simulink model "missile"  (R2018b)
settings: Solver=ode4  StartTime=0.0  StopTime=inf  FixedStep=0.03  RelTol=1e-3
values from neighbouring files (symbols this model uses):
  g = 9.8    [init.m]
  GP_switch = 1    [init.m]
  halfa_seeker_lock = 15    [init.m]
  init_m = [0 5000 0 180 0 deg2rad(0)]    [init.m]
  K = 3.5    [init.m]
  mass = [200 170 130]    [init.m]
  nn_lim = 40    [init.m]
  r_seeker_active = 20000    [init.m]
  S = 0.03    [init.m]
  TGO_max = 200    [init.m]
  thrust = [40000 20000 0]    [init.m]
  thrust_time_idx = [0 4 12]    [init.m]
undefined symbols (not defined in the file or in its folder): CD0, CDi, CL_idx, CLmax, ma_idx
libraries: aerolibasang x2, sharedutil x1, aerolibatmos2 x1, aerolibconvert2 x1
settings Model: Creator=niao4  LastModifiedBy=ysq
settings RTWCC: TargetLang=C++
settings GRTTargetCC: TargetLangStandard=C++03 (ISO)  MatFileLogging=off  MultiInstanceERTCode=on  CodeInterfacePackaging=C++ class

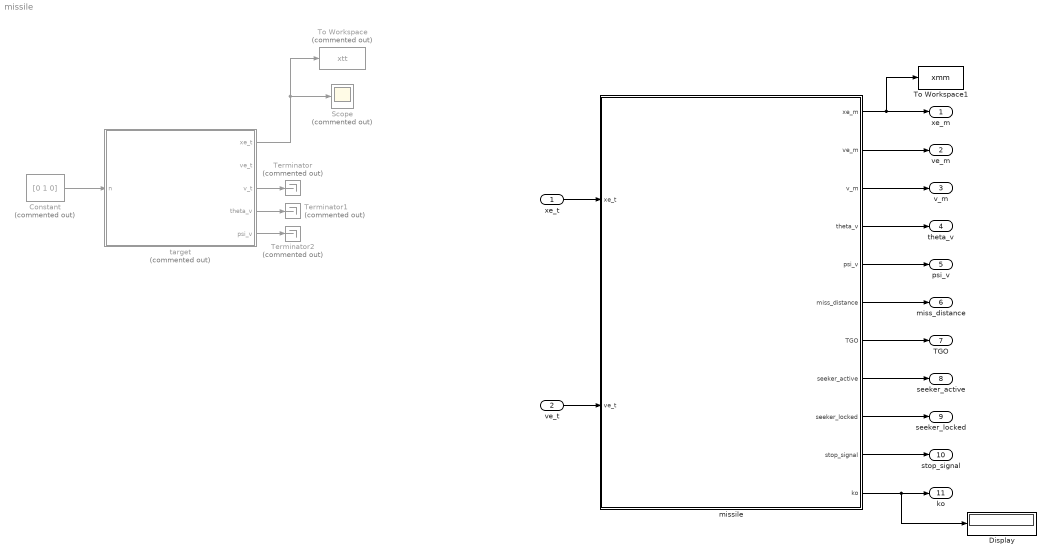
== system missile ==
  xe_t : Inport
  ve_t : Inport  Port=2
  Constant : Constant  Commented=on  Value=[0 1 0]
  Display : Display
  Scope : Scope  Commented=on
  Terminator : Terminator  Commented=on
  Terminator1 : Terminator  Commented=on
  Terminator2 : Terminator  Commented=on
  To Workspace : ToWorkspace  Commented=on  VariableName=xtt  SampleTime=-1
  To Workspace1 : ToWorkspace  VariableName=xmm  SampleTime=-1
  missile : Subsystem
  target : Subsystem  Commented=on
  xe_m : Outport
  ve_m : Outport  Port=2
  v_m : Outport  Port=3
  theta_v : Outport  Port=4
  psi_v : Outport  Port=5
  miss_distance : Outport  Port=6
  TGO : Outport  Port=7
  seeker_active : Outport  Port=8
  seeker_locked : Outport  Port=9
  stop_signal : Outport  Port=10
  ko : Outport  Port=11
  wires:
  target/5(psi_v) -> Terminator2/1
  Constant/1 -> target/1(n)
  target/4(theta_v) -> Terminator1/1
  target/3(v_t) -> Terminator/1
  target/1(xe_t) -> Scope/1, To Workspace/1
  missile/1(xe_m) -> To Workspace1/1, xe_m/1
  missile/2(ve_m) -> ve_m/1
  missile/3(v_m) -> v_m/1
  missile/4(theta_v) -> theta_v/1
  missile/5(psi_v) -> psi_v/1
  missile/6(miss_distance) -> miss_distance/1
  missile/7(TGO) -> TGO/1
  missile/8(seeker_active) -> seeker_active/1
  missile/9(seeker_locked) -> seeker_locked/1
  missile/10(stop_signal) -> stop_signal/1
  missile/11(ko) -> Display/1, ko/1
  xe_t/1 -> missile/1(xe_t)
  ve_t/1 -> missile/2(ve_t)

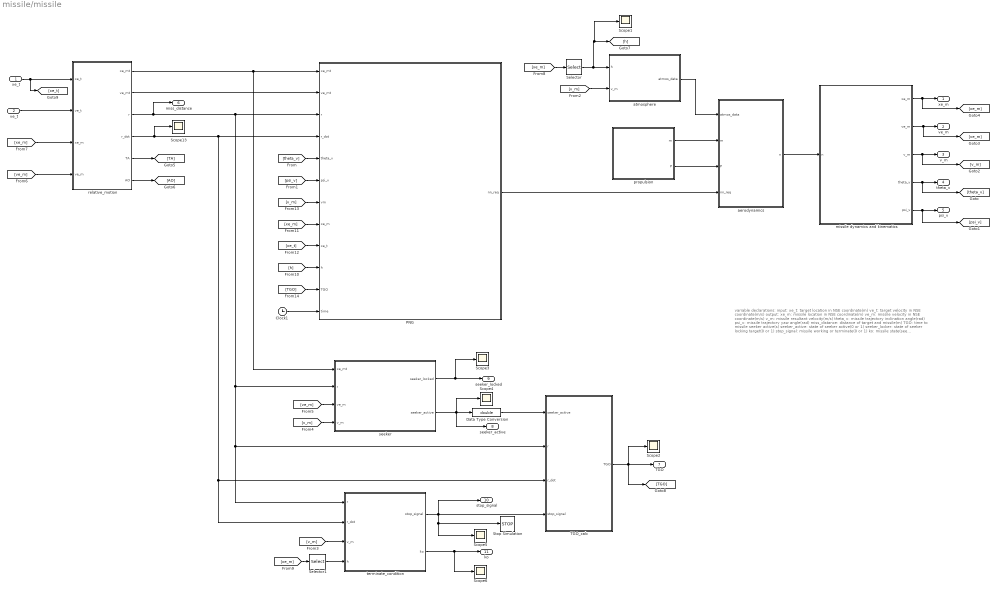
== system missile/missile ==
  note: variable declarations:
      | input:
      | xe_t: target location in NSE coordinate(m)
      | ve_t: target velocity in NSE coordinate(m/s)
      |
      | output:
      | xe_m: missile location in NSE coordinate(m)
      | ve_m: missile velocity in NSE coordinate(m/s)
      | v_m: missile resultant velocity(m/s)
      | theta_v: missile trajectory inclination angle(rad)
      | psi_v: missile trajectory yaw angle(rad)
      | miss_distance: distance of target and missile(m)
      | TGO: time to missile seeker active(s)
      | seeker_active: state of seeker active(0 or 1)
      | seeker_locker: state of seeker locking target(0 or 1)
      | stop_signal: missile working or terminate(0 or 1)
      | ko: missile state(see terminate_condition module for more)
      |
      | others:
      | xe_mt: relative location of missile and target in NSE coordinate(m)
      | ve_mt: relative velocity of missile and target in NSE coordinate(m/s)
      | r: same as miss_distance(m)
      | r_dot: closing rate of missile and target(m/s)
      | h: height of missile(m)
      | nn_req: request normal overload of missile calculated by PNG
      | n: actual tangential and normal overload of missile
      | m: mass of missile(kg)
      | P: propulsion of missile(N)
      | atmos_data: consist of mach and (kinetic pressure * reference area)
  xe_t : Inport
  ve_t : Inport  Port=2
  Clock1 : Clock
  Data Type Conversion : DataTypeConversion  OutDataTypeStr=double
  PNG : Subsystem
  Scope{1..6,13} (7 alike) : Scope
  Selector : Selector  InputPortWidth=3  IndexOptions=Index vector (dialog)  Indices=[2]  OutputSizes=1
  Selector1 : Selector  InputPortWidth=3  IndexOptions=Index vector (dialog)  Indices=[2]  OutputSizes=1
  Stop Simulation : Stop
  TGO_calc : Subsystem
  aerodynamics : Subsystem
  atmosphere : Subsystem
  missile dynamics and kinematics : Subsystem
  propulsion : Subsystem
  relative_motion : Subsystem
  seeker : Subsystem
  terminate_condition : Subsystem
  xe_m : Outport
  ve_m : Outport  Port=2
  v_m : Outport  Port=3
  theta_v : Outport  Port=4
  psi_v : Outport  Port=5
  miss_distance : Outport  Port=6
  TGO : Outport  Port=7
  seeker_active : Outport  Port=8
  seeker_locked : Outport  Port=9
  stop_signal : Outport  Port=10
  ko : Outport  Port=11
  wires:
  propulsion/2(P) -> aerodynamics/3(P)
  [v_m] -> terminate_condition/3(v_m)
  [xe_m] -> Selector/1
  xe_t/1 -> relative_motion/1(xe_t), [xe_t]
  propulsion/1(m) -> aerodynamics/2(m)
  Data Type Conversion/1 -> TGO_calc/1(seeker_active)
  missile dynamics and kinematics/1(xe_m) -> [xe_m], xe_m/1
  [xe_m] -> Selector1/1
  terminate_condition/1(stop_signal) -> stop_signal/1, Stop Simulation/1, Scope5/1, TGO_calc/4(stop_signal)
  seeker/2(seeker_active) -> seeker_active/1, Scope4/1, Data Type Conversion/1
  relative_motion/4(r_dot) -> terminate_condition/2(r_dot), TGO_calc/3(r_dot), PNG/4(r_dot), Scope13/1
  PNG/1(nn_req) -> aerodynamics/4(nn_req)
  relative_motion/5(TA) -> [TA]
  relative_motion/6(AO) -> [AO]
  missile dynamics and kinematics/2(ve_m) -> [ve_m], ve_m/1
  [v_m] -> seeker/4(v_m)
  missile dynamics and kinematics/3(v_m) -> [v_m], v_m/1
  seeker/1(seeker_locked) -> seeker_locked/1, Scope3/1
  terminate_condition/2(ko) -> ko/1, Scope6/1
  [ve_m] -> seeker/3(ve_m)
  missile dynamics and kinematics/4(theta_v) -> [theta_v], theta_v/1
  missile dynamics and kinematics/5(psi_v) -> [psi_v], psi_v/1
  relative_motion/1(xe_mt) -> seeker/1(xe_mt), PNG/1(xe_mt)
  TGO_calc/1(TGO) -> [TGO], TGO/1, Scope2/1
  [v_m] -> atmosphere/2(v_m)
  relative_motion/3(r) -> terminate_condition/1(r), TGO_calc/2(r), seeker/2(r), PNG/3(r), miss_distance/1
  atmosphere/1(atmos_data) -> aerodynamics/1(atmos_data)
  relative_motion/2(ve_mt) -> PNG/2(ve_mt)
  Selector/1 -> Scope1/1, [h], atmosphere/1(h)
  Selector1/1 -> terminate_condition/4(h)
  aerodynamics/1(n) -> missile dynamics and kinematics/1(n)
  [xe_m] -> PNG/8(xe_m)
  [xe_t] -> PNG/9(xe_t)
  [TGO] -> PNG/11(TGO)
  [v_m] -> PNG/7(vm)
  Clock1/1 -> PNG/12(time)
  [h] -> PNG/10(h)
  [psi_v] -> PNG/6(psi_v)
  [theta_v] -> PNG/5(theta_v)
  ve_t/1 -> relative_motion/2(ve_t)
  [xe_m] -> relative_motion/3(xe_m)
  [ve_m] -> relative_motion/4(ve_m)

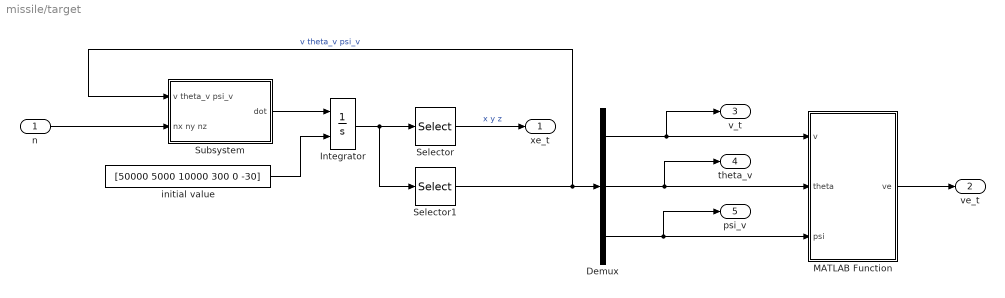
== system missile/target ==
  n : Inport
  Demux : Demux  Outputs=3
  Integrator : Integrator  InitialConditionSource=external
  MATLAB Function : MATLAB Function  TreatAsAtomicUnit=on
  Selector : Selector  InputPortWidth=6  IndexOptions=Index vector (dialog)  Indices=[1 2 3]  OutputSizes=1
  Selector1 : Selector  InputPortWidth=6  IndexOptions=Index vector (dialog)  Indices=[4 5 6]  OutputSizes=1
  Subsystem : Subsystem
  initial value : Constant  Value=[50000 5000 10000 300 0 -30]
  xe_t : Outport
  ve_t : Outport  Port=2
  v_t : Outport  Port=3
  theta_v : Outport  Port=4
  psi_v : Outport  Port=5
  wires:
  Selector/1 -> xe_t/1  "x y z"
  n/1 -> Subsystem/2(nx ny nz)
  Subsystem/1(dot) -> Integrator/1
  Integrator/1 -> Selector1/1, Selector/1
  Selector1/1 -> Subsystem/1(v theta_v psi_v), Demux/1  "v theta_v psi_v"
  initial value/1 -> Integrator/2
  MATLAB Function/1(ve) -> ve_t/1
  Demux/1 -> v_t/1, MATLAB Function/1(v)
  Demux/2 -> theta_v/1, MATLAB Function/2(theta)
  Demux/3 -> psi_v/1, MATLAB Function/3(psi)

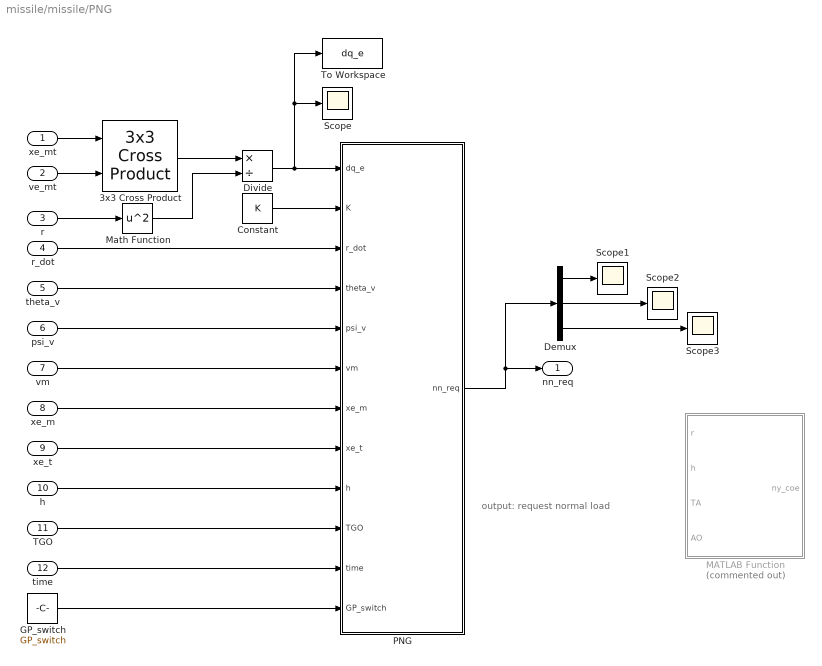
== system missile/missile/PNG ==
  note: output:
      | request normal load
  xe_mt : Inport
  ve_mt : Inport  Port=2
  r : Inport  Port=3
  r_dot : Inport  Port=4
  theta_v : Inport  Port=5
  psi_v : Inport  Port=6
  vm : Inport  Port=7
  xe_m : Inport  Port=8
  xe_t : Inport  Port=9
  h : Inport  Port=10
  TGO : Inport  Port=11
  time : Inport  Port=12
  3x3 Cross Product : sharedutil/3x3 Cross Product  aMode=aMode
      settings: SourceProductBaseCode=AE
  Constant : Constant  Value=K
  Demux : Demux  Outputs=3
  Divide : Product  Inputs=*/
  GP_switch : Constant  Value=GP_switch
  MATLAB Function : MATLAB Function  Commented=on  TreatAsAtomicUnit=on
  Math Function : Math  Operator=square  SaturateOnIntegerOverflow=on
  PNG : MATLAB Function  TreatAsAtomicUnit=on
  Scope{,1..3} (4 alike) : Scope
  To Workspace : ToWorkspace  VariableName=dq_e  SampleTime=-1
  nn_req : Outport
  wires:
  r/1 -> Math Function/1
  Math Function/1 -> Divide/2
  xe_mt/1 -> 3x3 Cross Product/1
  ve_mt/1 -> 3x3 Cross Product/2
  3x3 Cross Product/1 -> Divide/1
  PNG/1(nn_req) -> Demux/1, nn_req/1
  Divide/1 -> To Workspace/1, Scope/1, PNG/1(dq_e)
  r_dot/1 -> PNG/3(r_dot)
  theta_v/1 -> PNG/4(theta_v)
  psi_v/1 -> PNG/5(psi_v)
  Constant/1 -> PNG/2(K)
  Demux/1 -> Scope1/1
  Demux/2 -> Scope2/1
  Demux/3 -> Scope3/1
  time/1 -> PNG/11(time)
  vm/1 -> PNG/6(vm)
  TGO/1 -> PNG/10(TGO)
  h/1 -> PNG/9(h)
  xe_t/1 -> PNG/8(xe_t)
  xe_m/1 -> PNG/7(xe_m)
  GP_switch/1 -> PNG/12(GP_switch)

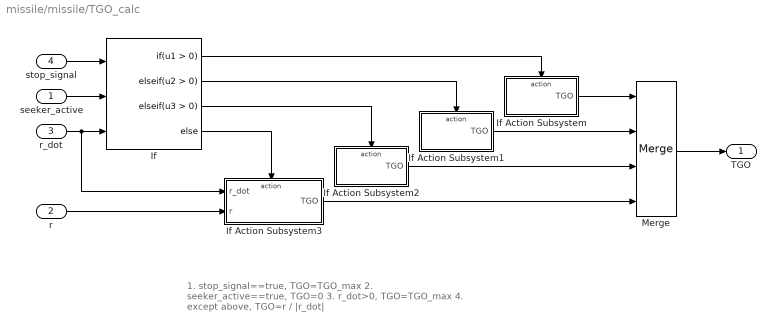
== system missile/missile/TGO_calc ==
  note: 1. stop_signal==true, TGO=TGO_max
      | 2. seeker_active==true, TGO=0
      | 3. r_dot>0, TGO=TGO_max
      | 4. except above, TGO=r / |r_dot|
  seeker_active : Inport
  r : Inport  Port=2
  r_dot : Inport  Port=3
  stop_signal : Inport  Port=4
  If : If  NumInputs=3  ElseIfExpressions=u2 > 0, u3 > 0
  If Action Subsystem : Subsystem  TreatAsAtomicUnit=on
  If Action Subsystem1 : Subsystem  TreatAsAtomicUnit=on
  If Action Subsystem2 : Subsystem  TreatAsAtomicUnit=on
  If Action Subsystem3 : Subsystem  TreatAsAtomicUnit=on
  Merge : Merge  Inputs=4
  TGO : Outport
  wires:
  If/3 -> If Action Subsystem2/Action
  stop_signal/1 -> If/1
  If/4 -> If Action Subsystem3/Action
  If Action Subsystem2/1(TGO) -> Merge/3
  If Action Subsystem/1(TGO) -> Merge/1
  If Action Subsystem1/1(TGO) -> Merge/2
  If/1 -> If Action Subsystem/Action
  r/1 -> If Action Subsystem3/2(r)
  seeker_active/1 -> If/2
  If Action Subsystem3/1(TGO) -> Merge/4
  If/2 -> If Action Subsystem1/Action
  r_dot/1 -> If Action Subsystem3/1(r_dot), If/3
  Merge/1 -> TGO/1

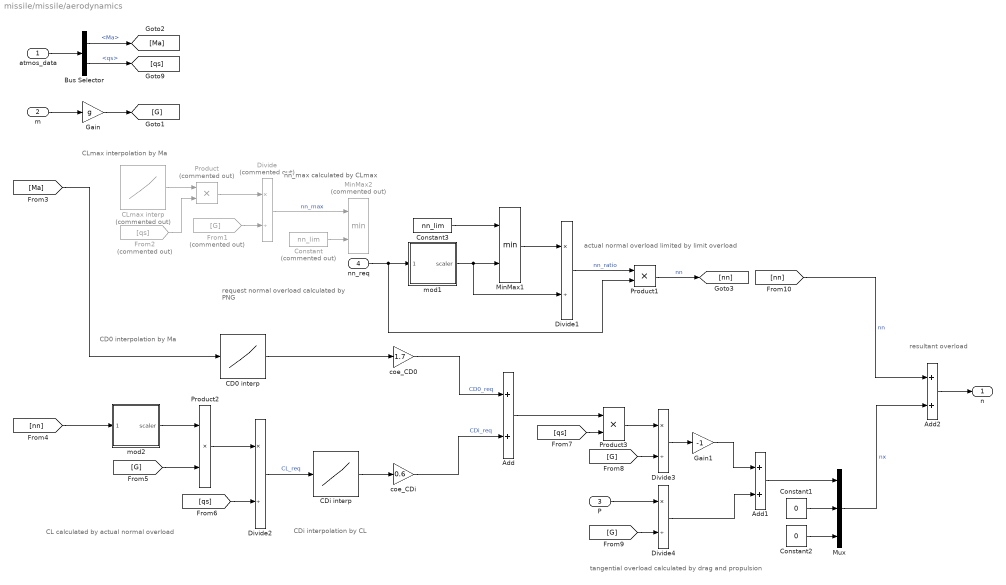
== system missile/missile/aerodynamics ==
  note: CD0 interpolation by Ma
  note: CDi interpolation by CL
  note: CLmax interpolation by Ma
  note: nn_max calculated by CLmax
  note: actual normal overload limited by limit overload
  note: CL calculated by actual normal overload
  note: tangential overload calculated by drag and propulsion
  note: resultant overload
  note: request normal overload
      | calculated by PNG
  atmos_data : Inport
  m : Inport  Port=2
  P : Inport  Port=3
  nn_req : Inport  Port=4
  Add : Sum
  Add1 : Sum
  Add2 : Sum
  Bus Selector : BusSelector  OutputSignals=Ma,qs
  CD0 interp : Lookup_n-D  NumberOfTableDimensions=1  BreakpointsForDimension1=ma_idx  Table=CD0  InternalRulePriority=Speed  RndMeth=Simplest  InputSameDT=on
  CDi interp : Lookup_n-D  NumberOfTableDimensions=1  BreakpointsForDimension1=CL_idx  Table=CDi  InternalRulePriority=Speed  RndMeth=Simplest  InputSameDT=on
  CLmax interp : Lookup_n-D  Commented=on  NumberOfTableDimensions=1  BreakpointsForDimension1=ma_idx  Table=CLmax  InternalRulePriority=Speed  RndMeth=Simplest  InputSameDT=on
  Constant : Constant  Commented=on  Value=nn_lim
  Constant1 : Constant  Value=0
  Constant2 : Constant  Value=0
  Constant3 : Constant  Value=nn_lim
  Divide : Product  Commented=on  Inputs=*/
  Divide{1..4} (4 alike) : Product  Inputs=*/
  From1 : From  Commented=on  GotoTag=G
  From2 : From  Commented=on  GotoTag=qs
  Gain : Gain  Gain=g
  Gain1 : Gain  Gain=-1
  MinMax1 : MinMax  Inputs=2
  MinMax2 : MinMax  Commented=on  Inputs=2
  Mux : Mux  Inputs=3
  Product : Product  Commented=on
  Product1 : Product
  Product2 : Product
  Product3 : Product
  coe_CD0 : Gain  Gain=1.7
  coe_CDi : Gain  Gain=0.6
  mod1 : Subsystem
  mod2 : Subsystem
  n : Outport
  wires:
  Divide4/1 -> Add1/2
  Gain1/1 -> Add1/1
  Product/1 -> Divide/1
  Add1/1 -> Mux/1
  From1/1 -> Divide/2
  [qs] -> Product3/2
  Divide1/1 -> Product1/1  "nn_ratio"
  Bus Selector/2 -> [qs]  "<qs>"
  [Ma] -> CD0 interp/1
  Divide3/1 -> Gain1/1
  mod2/1(scaler) -> Product2/1
  [G] -> Product2/2
  nn_req/1 -> Product1/2, mod1/1(vector)
  m/1 -> Gain/1
  Product3/1 -> Divide3/1
  Divide2/1 -> CDi interp/1  "CL_req"
  Divide/1 -> MinMax2/1  "nn_max"
  CLmax interp/1 -> Product/1
  [G] -> Divide3/2
  atmos_data/1 -> Bus Selector/1
  Gain/1 -> [G]
  P/1 -> Divide4/1
  Constant/1 -> MinMax2/2
  MinMax1/1 -> Divide1/1
  Add2/1 -> n/1
  Product2/1 -> Divide2/1
  Add/1 -> Product3/1
  Constant2/1 -> Mux/3
  Constant1/1 -> Mux/2
  [nn] -> mod2/1(vector)
  Bus Selector/1 -> [Ma]  "<Ma>"
  From2/1 -> Product/2
  [qs] -> Divide2/2
  [G] -> Divide4/2
  Mux/1 -> Add2/2  "nx"
  Product1/1 -> [nn]  "nn"
  [nn] -> Add2/1  "nn"
  CD0 interp/1 -> coe_CD0/1
  CDi interp/1 -> coe_CDi/1
  coe_CD0/1 -> Add/1  "CD0_req"
  coe_CDi/1 -> Add/2  "CDi_req"
  mod1/1(scaler) -> Divide1/2, MinMax1/2
  Constant3/1 -> MinMax1/1

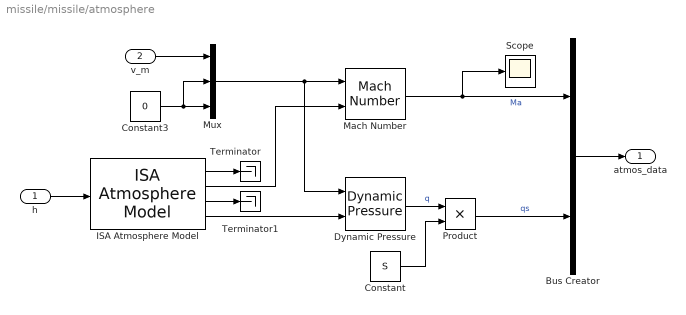
== system missile/missile/atmosphere ==
  h : Inport
  v_m : Inport  Port=2
  Bus Creator : BusCreator  Inputs=2
  Constant : Constant  Value=S
  Constant3 : Constant  Value=0
  Dynamic Pressure : aerolibasang/Dynamic Pressure
  ISA Atmosphere Model : aerolibatmos2/ISA Atmosphere Model  custom=off  g=9.80665  gamma=1.4  R=287.0531  L=0.0065  h_trop=11000  h_strat=20000  rho0=1.225  P0=101325  T0=288.15  h0=0
      settings: SourceProductName=Aerospace Blockset
  Mach Number : aerolibasang/Mach Number
      settings: SourceProductName=Aerospace Blockset  SourceProductBaseCode=AE
  Mux : Mux  Inputs=3
  Product : Product
  Scope : Scope
  Terminator : Terminator
  Terminator1 : Terminator
  atmos_data : Outport
  wires:
  ISA Atmosphere Model/1 -> Terminator/1
  Bus Creator/1 -> atmos_data/1
  Constant3/1 -> Mux/2, Mux/3
  v_m/1 -> Mux/1
  ISA Atmosphere Model/2 -> Mach Number/2
  Mux/1 -> Dynamic Pressure/1, Mach Number/1
  ISA Atmosphere Model/4 -> Dynamic Pressure/2
  ISA Atmosphere Model/3 -> Terminator1/1
  h/1 -> ISA Atmosphere Model/1
  Dynamic Pressure/1 -> Product/1  "q"
  Constant/1 -> Product/2
  Product/1 -> Bus Creator/2  "qs"
  Mach Number/1 -> Scope/1, Bus Creator/1  "Ma"

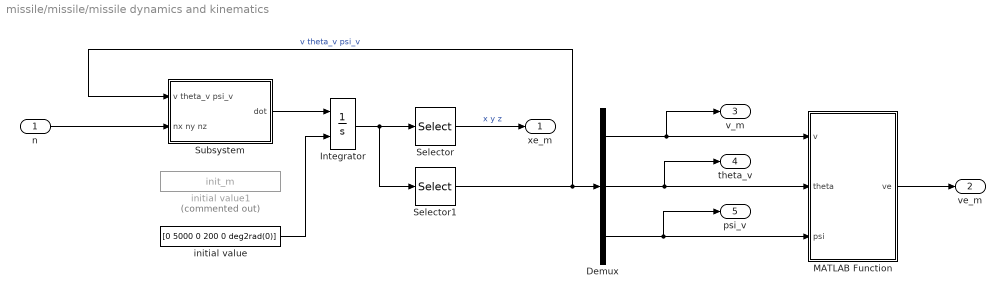
== system missile/missile/missile dynamics and kinematics ==
  n : Inport  PortDimensions=3
  Demux : Demux  Outputs=3
  Integrator : Integrator  InitialConditionSource=external
  MATLAB Function : MATLAB Function  TreatAsAtomicUnit=on
  Selector : Selector  InputPortWidth=6  IndexOptions=Index vector (dialog)  Indices=[1 2 3]  OutputSizes=1
  Selector1 : Selector  InputPortWidth=6  IndexOptions=Index vector (dialog)  Indices=[4 5 6]  OutputSizes=1
  Subsystem : Subsystem
  initial value : Constant  Value=[0 5000 0 200 0 deg2rad(0)]
  initial value1 : Constant  Commented=on  Value=init_m
  xe_m : Outport
  ve_m : Outport  Port=2
  v_m : Outport  Port=3
  theta_v : Outport  Port=4
  psi_v : Outport  Port=5
  wires:
  Integrator/1 -> Selector1/1, Selector/1
  Demux/1 -> v_m/1, MATLAB Function/1(v)
  n/1 -> Subsystem/2(nx ny nz)
  Demux/2 -> theta_v/1, MATLAB Function/2(theta)
  Subsystem/1(dot) -> Integrator/1
  MATLAB Function/1(ve) -> ve_m/1
  Selector1/1 -> Subsystem/1(v theta_v psi_v), Demux/1  "v theta_v psi_v"
  Selector/1 -> xe_m/1  "x y z"
  Demux/3 -> psi_v/1, MATLAB Function/3(psi)
  initial value/1 -> Integrator/2

== system missile/missile/propulsion ==
  Clock : Clock
  mass Lookup Table1 : Lookup_n-D  NumberOfTableDimensions=1  BreakpointsForDimension1=thrust_time_idx  IndexSearchMethod=Linear search  BeginIndexSearchUsingPreviousIndexResult=on  Table=mass  InterpMethod=Flat  InternalRulePriority=Speed  RndMeth=Simplest  InputSameDT=on
  thrust Lookup Table : Lookup_n-D  NumberOfTableDimensions=1  BreakpointsForDimension1=thrust_time_idx  IndexSearchMethod=Linear search  BeginIndexSearchUsingPreviousIndexResult=on  Table=thrust  InterpMethod=Flat  InternalRulePriority=Speed  RndMeth=Simplest  InputSameDT=on
  m : Outport
  P : Outport  Port=2
  wires:
  Clock/1 -> thrust Lookup Table/1, mass Lookup Table1/1
  thrust Lookup Table/1 -> P/1
  mass Lookup Table1/1 -> m/1

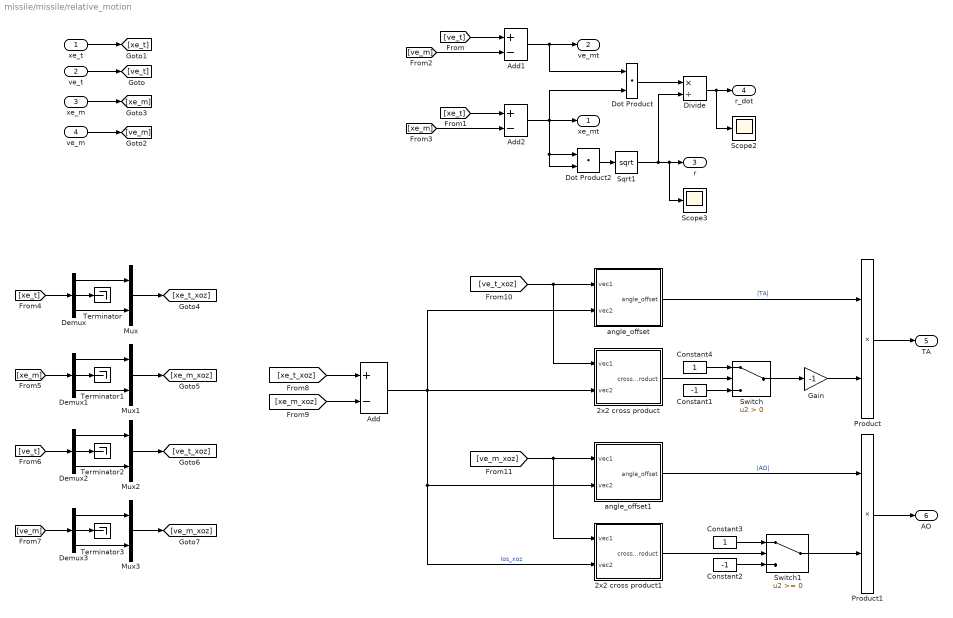
== system missile/missile/relative_motion ==
  xe_t : Inport
  ve_t : Inport  Port=2
  xe_m : Inport  Port=3
  ve_m : Inport  Port=4
  2x2 cross product : Subsystem
  2x2 cross product1 : Subsystem
  Add : Sum  Inputs=+-
  Add1 : Sum  Inputs=+-
  Add2 : Sum  Inputs=+-
  Constant1 : Constant  Value=-1
  Constant2 : Constant  Value=-1
  Constant3 : Constant
  Constant4 : Constant
  Demux{,1..3} (4 alike) : Demux  Outputs=3
  Divide : Product  Inputs=*/
  Dot Product : DotProduct  InputSameDT=on  OutDataTypeStr=Inherit: Inherit via internal rule
  Dot Product2 : DotProduct  InputSameDT=on  OutDataTypeStr=Inherit: Inherit via internal rule
  Gain : Gain  Gain=-1
  Mux{,1..3} (4 alike) : Mux  Inputs=2
  Product : Product
  Product1 : Product
  Scope2 : Scope
  Scope3 : Scope
  Sqrt1 : Sqrt  SaturateOnIntegerOverflow=on
  Switch : Switch  Criteria=u2 > Threshold
  Switch1 : Switch
  Terminator{,1..3} (4 alike) : Terminator
  angle_offset : Subsystem
  angle_offset1 : Subsystem
  xe_mt : Outport
  ve_mt : Outport  Port=2
  r : Outport  Port=3
  r_dot : Outport  Port=4
  TA : Outport  Port=5
  AO : Outport  Port=6
  wires:
  Dot Product2/1 -> Sqrt1/1
  Add2/1 -> Dot Product/2, Dot Product2/2, Dot Product2/1, xe_mt/1
  Sqrt1/1 -> Scope3/1, r/1, Divide/2
  Add1/1 -> Dot Product/1, ve_mt/1
  Dot Product/1 -> Divide/1
  Divide/1 -> Scope2/1, r_dot/1
  Demux/2 -> Terminator/1
  Demux/1 -> Mux/1
  Demux/3 -> Mux/2
  ve_t/1 -> [ve_t]
  [ve_t] -> Add1/1
  ve_m/1 -> [ve_m]
  [ve_m] -> Add1/2
  xe_t/1 -> [xe_t]
  [xe_t] -> Add2/1
  xe_m/1 -> [xe_m]
  [xe_m] -> Add2/2
  [xe_t] -> Demux/1
  [xe_m] -> Demux1/1
  Demux1/3 -> Mux1/2
  Demux1/1 -> Mux1/1
  Demux1/2 -> Terminator1/1
  Mux/1 -> [xe_t_xoz]
  Mux1/1 -> [xe_m_xoz]
  Mux3/1 -> [ve_m_xoz]
  Mux2/1 -> [ve_t_xoz]
  Demux3/2 -> Terminator3/1
  Demux3/1 -> Mux3/1
  Demux3/3 -> Mux3/2
  [ve_m] -> Demux3/1
  [ve_t] -> Demux2/1
  Demux2/3 -> Mux2/2
  Demux2/1 -> Mux2/1
  Demux2/2 -> Terminator2/1
  [xe_t_xoz] -> Add/1
  [xe_m_xoz] -> Add/2
  Add/1 -> angle_offset/2(vec2), 2x2 cross product/2(vec2), angle_offset1/2(vec2), 2x2 cross product1/2(vec2)  "los_xoz"
  [ve_t_xoz] -> 2x2 cross product/1(vec1), angle_offset/1(vec1)
  Gain/1 -> Product/2
  angle_offset/1(angle_offset) -> Product/1  "|TA|"
  Product/1 -> TA/1
  Product1/1 -> AO/1
  angle_offset1/1(angle_offset) -> Product1/1  "|AO|"
  [ve_m_xoz] -> angle_offset1/1(vec1), 2x2 cross product1/1(vec1)
  Constant4/1 -> Switch/1
  Switch/1 -> Gain/1
  2x2 cross product/1(crossproduct) -> Switch/2
  Constant1/1 -> Switch/3
  Constant3/1 -> Switch1/1
  Constant2/1 -> Switch1/3
  Switch1/1 -> Product1/2
  2x2 cross product1/1(crossproduct) -> Switch1/2

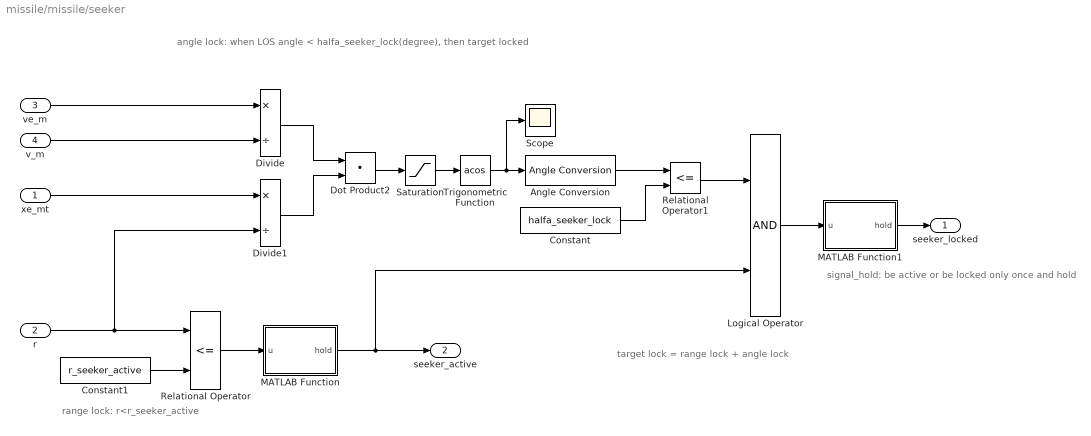
== system missile/missile/seeker ==
  note: target lock = range lock + angle lock
  note: signal_hold:
      | be active or be locked only once and hold
  note: range lock:
      | r<r_seeker_active
  note: angle lock:
      | when LOS angle < halfa_seeker_lock(degree), then target locked
  xe_mt : Inport
  r : Inport  Port=2
  ve_m : Inport  Port=3
  v_m : Inport  Port=4
  Angle Conversion : aerolibconvert2/Angle Conversion  IU=rad  OU=deg
  Constant : Constant  Value=halfa_seeker_lock
  Constant1 : Constant  Value=r_seeker_active
  Divide : Product  Inputs=*/
  Divide1 : Product  Inputs=*/
  Dot Product2 : DotProduct  InputSameDT=on  OutDataTypeStr=Inherit: Inherit via internal rule
  Logical Operator : Logic  AllPortsSameDT=off  OutDataTypeStr=boolean
  MATLAB Function : MATLAB Function  TreatAsAtomicUnit=on
  MATLAB Function1 : MATLAB Function  TreatAsAtomicUnit=on
  Relational Operator : RelationalOperator  Operator=<=  OutDataTypeStr=boolean  RndMeth=Simplest
  Relational Operator1 : RelationalOperator  Operator=<=  OutDataTypeStr=boolean  RndMeth=Simplest
  Saturation : Saturate  UpperLimit=1  LowerLimit=-1
  Scope : Scope
  Trigonometric Function : Trigonometry  Operator=acos
  seeker_locked : Outport
  seeker_active : Outport  Port=2
  wires:
  Relational Operator/1 -> MATLAB Function/1(u)
  Constant1/1 -> Relational Operator/2
  ve_m/1 -> Divide/1
  xe_mt/1 -> Divide1/1
  Divide/1 -> Dot Product2/1
  Divide1/1 -> Dot Product2/2
  Trigonometric Function/1 -> Scope/1, Angle Conversion/1
  Angle Conversion/1 -> Relational Operator1/1
  Constant/1 -> Relational Operator1/2
  MATLAB Function/1(hold) -> Logical Operator/2, seeker_active/1
  r/1 -> Divide1/2, Relational Operator/1
  Relational Operator1/1 -> Logical Operator/1
  Logical Operator/1 -> MATLAB Function1/1(u)
  MATLAB Function1/1(hold) -> seeker_locked/1
  v_m/1 -> Divide/2
  Dot Product2/1 -> Saturation/1
  Saturation/1 -> Trigonometric Function/1

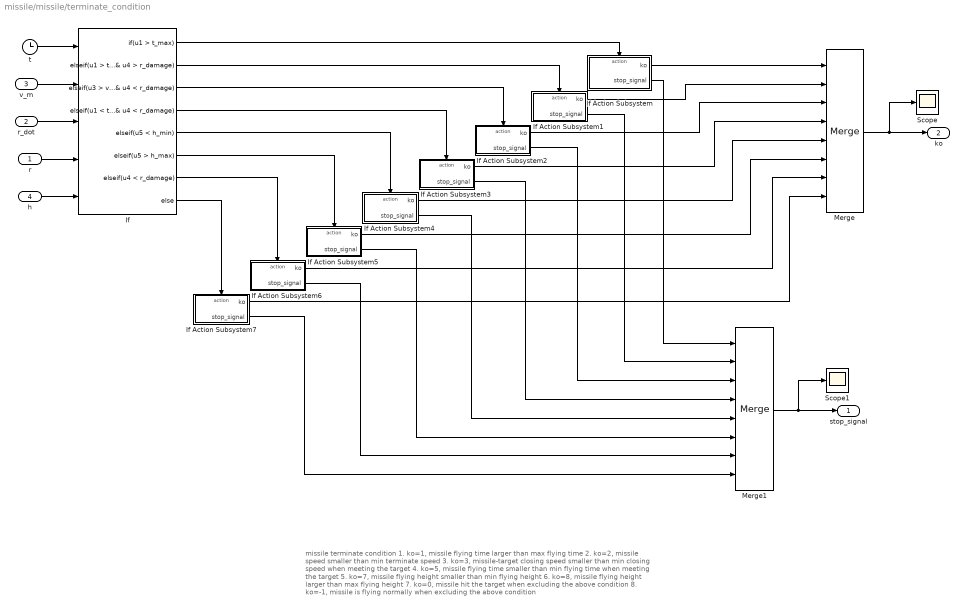
== system missile/missile/terminate_condition ==
  note: missile terminate condition
      | 1. ko=1, missile flying time larger than max flying time
      | 2. ko=2, missile speed smaller than min terminate speed
      | 3. ko=3, missile-target closing speed smaller than min closing speed when meeting the target
      | 4. ko=5, missile flying time smaller than min flying time when meeting the target
      | 5. ko=7, missile flying height smaller than min flying height
      | 6. ko=8, missile flying height larger than max flying height
      | 7. ko=0, missile hit the target when excluding the above condition
      | 8. ko=-1, missile is flying normally when excluding the above condition
  r : Inport
  r_dot : Inport  Port=2
  v_m : Inport  Port=3
  h : Inport  Port=4
  If : If  NumInputs=5  IfExpression=u1 > t_max  ElseIfExpressions=u1 > thrust_time_idx(3) & u2 < vm_term & u4 > r_damage, u3 > vmt_term & u4 < r_damage, u1 < t_min & u4 < r_damage, u5 < h_min, u5 > h_max, u4 < r_damage
  If Action Subsystem : Subsystem  TreatAsAtomicUnit=on
  If Action Subsystem1 : Subsystem  TreatAsAtomicUnit=on
  If Action Subsystem2 : Subsystem  TreatAsAtomicUnit=on
  If Action Subsystem3 : Subsystem  TreatAsAtomicUnit=on
  If Action Subsystem4 : Subsystem  TreatAsAtomicUnit=on
  If Action Subsystem5 : Subsystem  TreatAsAtomicUnit=on
  If Action Subsystem6 : Subsystem  TreatAsAtomicUnit=on
  If Action Subsystem7 : Subsystem  TreatAsAtomicUnit=on
  Merge : Merge  Inputs=8
  Merge1 : Merge  Inputs=8
  Scope : Scope
  Scope1 : Scope
  t : Clock
  stop_signal : Outport
  ko : Outport  Port=2
  wires:
  If Action Subsystem7/2(stop_signal) -> Merge1/8
  If/3 -> If Action Subsystem2/Action
  v_m/1 -> If/2
  If/7 -> If Action Subsystem6/Action
  h/1 -> If/5
  If Action Subsystem4/1(ko) -> Merge/5
  r/1 -> If/4
  If/8 -> If Action Subsystem7/Action
  t/1 -> If/1
  If Action Subsystem5/1(ko) -> Merge/6
  If Action Subsystem/1(ko) -> Merge/1
  Merge/1 -> ko/1, Scope/1
  If/4 -> If Action Subsystem3/Action
  If Action Subsystem6/2(stop_signal) -> Merge1/7
  If Action Subsystem5/2(stop_signal) -> Merge1/6
  If Action Subsystem4/2(stop_signal) -> Merge1/5
  r_dot/1 -> If/3
  If Action Subsystem2/1(ko) -> Merge/3
  If/6 -> If Action Subsystem5/Action
  If Action Subsystem7/1(ko) -> Merge/8
  If Action Subsystem1/2(stop_signal) -> Merge1/2
  If Action Subsystem2/2(stop_signal) -> Merge1/3
  Merge1/1 -> stop_signal/1, Scope1/1
  If Action Subsystem6/1(ko) -> Merge/7
  If/2 -> If Action Subsystem1/Action
  If/5 -> If Action Subsystem4/Action
  If Action Subsystem3/1(ko) -> Merge/4
  If/1 -> If Action Subsystem/Action
  If Action Subsystem3/2(stop_signal) -> Merge1/4
  If Action Subsystem1/1(ko) -> Merge/2
  If Action Subsystem/2(stop_signal) -> Merge1/1

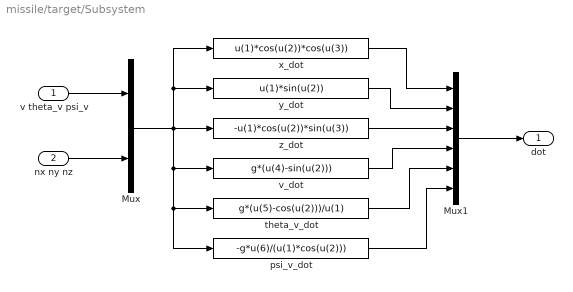
== system missile/target/Subsystem ==
  v theta_v psi_v : Inport
  nx ny nz : Inport  Port=2
  Mux : Mux  Inputs=2
  Mux1 : Mux  Inputs=6
  psi_v_dot : Fcn  Expr=-g*u(6)/(u(1)*cos(u(2)))
  theta_v_dot : Fcn  Expr=g*(u(5)-cos(u(2)))/u(1)
  v_dot : Fcn  Expr=g*(u(4)-sin(u(2)))
  x_dot : Fcn  Expr=u(1)*cos(u(2))*cos(u(3))
  y_dot : Fcn  Expr=u(1)*sin(u(2))
  z_dot : Fcn  Expr=-u(1)*cos(u(2))*sin(u(3))
  dot : Outport
  wires:
  theta_v_dot/1 -> Mux1/5
  psi_v_dot/1 -> Mux1/6
  Mux1/1 -> dot/1
  y_dot/1 -> Mux1/2
  Mux/1 -> psi_v_dot/1, theta_v_dot/1, v_dot/1, y_dot/1, x_dot/1, z_dot/1
  x_dot/1 -> Mux1/1
  v_dot/1 -> Mux1/4
  z_dot/1 -> Mux1/3
  nx ny nz/1 -> Mux/2
  v theta_v psi_v/1 -> Mux/1

== system missile/missile/TGO_calc/If Action Subsystem ==
  Action Port : ActionPort  ActionType=then
  TGO_max : Constant  Value=TGO_max
  TGO : Outport
  wires:
  TGO_max/1 -> TGO/1

== system missile/missile/TGO_calc/If Action Subsystem1 ==
  Action Port : ActionPort  ActionType=elseif
  Constant : Constant  Value=0
  TGO : Outport
  wires:
  Constant/1 -> TGO/1

== system missile/missile/TGO_calc/If Action Subsystem2 ==
  Action Port : ActionPort  ActionType=elseif
  TGO_max : Constant  Value=TGO_max
  TGO : Outport
  wires:
  TGO_max/1 -> TGO/1

== system missile/missile/TGO_calc/If Action Subsystem3 ==
  r_dot : Inport
  r : Inport  Port=2
  Action Port : ActionPort  ActionType=else
  Abs : Abs
  Divide : Product  Inputs=*/
  Saturation : Saturate  UpperLimit=200  LowerLimit=0
  Saturation1 : Saturate  UpperLimit=10000  LowerLimit=0.001
  TGO : Outport
  wires:
  r/1 -> Divide/1
  r_dot/1 -> Abs/1
  Divide/1 -> Saturation/1
  Saturation/1 -> TGO/1
  Abs/1 -> Saturation1/1
  Saturation1/1 -> Divide/2

== system missile/missile/aerodynamics/mod1 ==
  vector : Inport
  Dot Product : DotProduct  InputSameDT=on  OutDataTypeStr=Inherit: Inherit via internal rule
  Sqrt : Sqrt  SaturateOnIntegerOverflow=on
  scaler : Outport
  wires:
  vector/1 -> Dot Product/2, Dot Product/1
  Sqrt/1 -> scaler/1
  Dot Product/1 -> Sqrt/1

== system missile/missile/aerodynamics/mod2 ==
  vector : Inport
  Dot Product : DotProduct  InputSameDT=on  OutDataTypeStr=Inherit: Inherit via internal rule
  Sqrt : Sqrt  SaturateOnIntegerOverflow=on
  scaler : Outport
  wires:
  Dot Product/1 -> Sqrt/1
  Sqrt/1 -> scaler/1
  vector/1 -> Dot Product/1, Dot Product/2

== system missile/missile/missile dynamics and kinematics/Subsystem ==
  note: differential equation:
      | dx/dt = v*cos(theta_v)*cos(psi_v)
      | dy/dt = v*sin(theta_v)
      | dz/dt = -v*cos(theta_v)*sin(psi_v)
      | dv/dt = g*(nx-sin(theta_v))
      | dtheta_v/dt = g*(ny-cos(theta_v))/v
      | dpsi_v/dt = -g*nz/(v*cos(theta_v))
  v theta_v psi_v : Inport
  nx ny nz : Inport  Port=2
  Mux : Mux  Inputs=2
  Mux1 : Mux  Inputs=6
  psi_v_dot : Fcn  Expr=-g*u(6)/(u(1)*cos(u(2)))
  theta_v_dot : Fcn  Expr=g*(u(5)-cos(u(2)))/u(1)
  v_dot : Fcn  Expr=g*(u(4)-sin(u(2)))
  x_dot : Fcn  Expr=u(1)*cos(u(2))*cos(u(3))
  y_dot : Fcn  Expr=u(1)*sin(u(2))
  z_dot : Fcn  Expr=-u(1)*cos(u(2))*sin(u(3))
  dot : Outport
  wires:
  theta_v_dot/1 -> Mux1/5
  psi_v_dot/1 -> Mux1/6
  Mux1/1 -> dot/1
  y_dot/1 -> Mux1/2
  Mux/1 -> psi_v_dot/1, theta_v_dot/1, v_dot/1, y_dot/1, x_dot/1, z_dot/1
  x_dot/1 -> Mux1/1
  v_dot/1 -> Mux1/4
  z_dot/1 -> Mux1/3
  nx ny nz/1 -> Mux/2
  v theta_v psi_v/1 -> Mux/1

== system missile/missile/relative_motion/2x2 cross product ==
  vec1 : Inport
  vec2 : Inport  Port=2
  Demux : Demux  Outputs=2
  Demux1 : Demux  Outputs=2
  Product : Product
  Product1 : Product
  Subtract : Sum  Inputs=+-
  vec_normalize : Subsystem
  vec_normalize1 : Subsystem
  crossproduct : Outport
  wires:
  Subtract/1 -> crossproduct/1
  Product1/1 -> Subtract/2
  Product/1 -> Subtract/1
  vec_normalize/1(unit_vec) -> Demux1/1
  vec_normalize1/1(unit_vec) -> Demux/1
  vec2/1 -> vec_normalize/1(vec)
  vec1/1 -> vec_normalize1/1(vec)
  Demux/2 -> Product/1
  Demux1/1 -> Product/2
  Demux/1 -> Product1/1
  Demux1/2 -> Product1/2

== system missile/missile/relative_motion/2x2 cross product1 ==
  vec1 : Inport
  vec2 : Inport  Port=2
  Demux : Demux  Outputs=2
  Demux1 : Demux  Outputs=2
  Product : Product
  Product1 : Product
  Subtract : Sum  Inputs=+-
  vec_normalize : Subsystem
  vec_normalize1 : Subsystem
  crossproduct : Outport
  wires:
  Demux1/2 -> Product1/2
  Demux/1 -> Product1/1
  Demux1/1 -> Product/2
  Demux/2 -> Product/1
  vec1/1 -> vec_normalize1/1(vec)
  vec2/1 -> vec_normalize/1(vec)
  vec_normalize1/1(unit_vec) -> Demux/1
  vec_normalize/1(unit_vec) -> Demux1/1
  Product/1 -> Subtract/1
  Product1/1 -> Subtract/2
  Subtract/1 -> crossproduct/1

== system missile/missile/relative_motion/angle_offset ==
  vec1 : Inport
  vec2 : Inport  Port=2
  Dot Product : DotProduct  InputSameDT=on  OutDataTypeStr=Inherit: Inherit via internal rule
  Saturation : Saturate  UpperLimit=1  LowerLimit=-1
  Trigonometric Function : Trigonometry  Operator=acos
  vec_normalize : Subsystem
  vec_normalize1 : Subsystem
  angle_offset : Outport
  wires:
  Trigonometric Function/1 -> angle_offset/1
  vec2/1 -> vec_normalize/1(vec)
  Dot Product/1 -> Saturation/1
  vec1/1 -> vec_normalize1/1(vec)
  vec_normalize/1(unit_vec) -> Dot Product/2
  vec_normalize1/1(unit_vec) -> Dot Product/1
  Saturation/1 -> Trigonometric Function/1

== system missile/missile/relative_motion/angle_offset1 ==
  vec1 : Inport
  vec2 : Inport  Port=2
  Dot Product : DotProduct  InputSameDT=on  OutDataTypeStr=Inherit: Inherit via internal rule
  Saturation : Saturate  UpperLimit=1  LowerLimit=-1
  Trigonometric Function : Trigonometry  Operator=acos
  vec_normalize : Subsystem
  vec_normalize1 : Subsystem
  angle_offset : Outport
  wires:
  Saturation/1 -> Trigonometric Function/1
  vec_normalize1/1(unit_vec) -> Dot Product/1
  vec_normalize/1(unit_vec) -> Dot Product/2
  vec1/1 -> vec_normalize1/1(vec)
  Dot Product/1 -> Saturation/1
  vec2/1 -> vec_normalize/1(vec)
  Trigonometric Function/1 -> angle_offset/1

== system missile/missile/terminate_condition/If Action Subsystem ==
  Action Port : ActionPort  ActionType=then
  Constant : Constant
  Constant1 : Constant
  ko : Outport
  stop_signal : Outport  Port=2
  wires:
  Constant/1 -> ko/1
  Constant1/1 -> stop_signal/1

== system missile/missile/terminate_condition/If Action Subsystem1 ==
  Action Port : ActionPort  ActionType=elseif
  Constant : Constant  Value=2
  Constant1 : Constant
  ko : Outport
  stop_signal : Outport  Port=2
  wires:
  Constant/1 -> ko/1
  Constant1/1 -> stop_signal/1

== system missile/missile/terminate_condition/If Action Subsystem2 ==
  Action Port : ActionPort  ActionType=elseif
  Constant : Constant  Value=3
  Constant1 : Constant
  ko : Outport
  stop_signal : Outport  Port=2
  wires:
  Constant1/1 -> stop_signal/1
  Constant/1 -> ko/1

== system missile/missile/terminate_condition/If Action Subsystem3 ==
  Action Port : ActionPort  ActionType=elseif
  Constant : Constant  Value=5
  Constant1 : Constant
  ko : Outport
  stop_signal : Outport  Port=2
  wires:
  Constant/1 -> ko/1
  Constant1/1 -> stop_signal/1

== system missile/missile/terminate_condition/If Action Subsystem4 ==
  Action Port : ActionPort  ActionType=elseif
  Constant : Constant  Value=7
  Constant1 : Constant
  ko : Outport
  stop_signal : Outport  Port=2
  wires:
  Constant1/1 -> stop_signal/1
  Constant/1 -> ko/1

== system missile/missile/terminate_condition/If Action Subsystem5 ==
  Action Port : ActionPort  ActionType=elseif
  Constant : Constant  Value=8
  Constant1 : Constant
  ko : Outport
  stop_signal : Outport  Port=2
  wires:
  Constant/1 -> ko/1
  Constant1/1 -> stop_signal/1

== system missile/missile/terminate_condition/If Action Subsystem6 ==
  Action Port : ActionPort  ActionType=elseif
  Constant : Constant  Value=0
  Constant1 : Constant
  ko : Outport
  stop_signal : Outport  Port=2
  wires:
  Constant1/1 -> stop_signal/1
  Constant/1 -> ko/1

== system missile/missile/terminate_condition/If Action Subsystem7 ==
  Action Port : ActionPort  ActionType=else
  Constant : Constant  Value=-1
  Constant1 : Constant  Value=0
  ko : Outport
  stop_signal : Outport  Port=2
  wires:
  Constant/1 -> ko/1
  Constant1/1 -> stop_signal/1

== system missile/missile/relative_motion/2x2 cross product/vec_normalize ==
  vec : Inport
  Divide : Product  Inputs=*/
  vec_length : Subsystem
  unit_vec : Outport
  wires:
  vec/1 -> vec_length/1(vec), Divide/1
  Divide/1 -> unit_vec/1
  vec_length/1(scaler) -> Divide/2

== system missile/missile/relative_motion/2x2 cross product/vec_normalize1 ==
  vec : Inport
  Divide : Product  Inputs=*/
  vec_length : Subsystem
  unit_vec : Outport
  wires:
  vec_length/1(scaler) -> Divide/2
  Divide/1 -> unit_vec/1
  vec/1 -> Divide/1, vec_length/1(vec)

== system missile/missile/relative_motion/2x2 cross product1/vec_normalize ==
  vec : Inport
  Divide : Product  Inputs=*/
  vec_length : Subsystem
  unit_vec : Outport
  wires:
  vec_length/1(scaler) -> Divide/2
  Divide/1 -> unit_vec/1
  vec/1 -> Divide/1, vec_length/1(vec)

== system missile/missile/relative_motion/2x2 cross product1/vec_normalize1 ==
  vec : Inport
  Divide : Product  Inputs=*/
  vec_length : Subsystem
  unit_vec : Outport
  wires:
  vec/1 -> vec_length/1(vec), Divide/1
  Divide/1 -> unit_vec/1
  vec_length/1(scaler) -> Divide/2

== system missile/missile/relative_motion/angle_offset/vec_normalize ==
  vec : Inport
  Divide : Product  Inputs=*/
  vec_length : Subsystem
  unit_vec : Outport
  wires:
  vec/1 -> vec_length/1(vec), Divide/1
  Divide/1 -> unit_vec/1
  vec_length/1(scaler) -> Divide/2

== system missile/missile/relative_motion/angle_offset/vec_normalize1 ==
  vec : Inport
  Divide : Product  Inputs=*/
  vec_length : Subsystem
  unit_vec : Outport
  wires:
  vec_length/1(scaler) -> Divide/2
  Divide/1 -> unit_vec/1
  vec/1 -> Divide/1, vec_length/1(vec)

== system missile/missile/relative_motion/angle_offset1/vec_normalize ==
  vec : Inport
  Divide : Product  Inputs=*/
  vec_length : Subsystem
  unit_vec : Outport
  wires:
  vec_length/1(scaler) -> Divide/2
  Divide/1 -> unit_vec/1
  vec/1 -> Divide/1, vec_length/1(vec)

== system missile/missile/relative_motion/angle_offset1/vec_normalize1 ==
  vec : Inport
  Divide : Product  Inputs=*/
  vec_length : Subsystem
  unit_vec : Outport
  wires:
  vec/1 -> vec_length/1(vec), Divide/1
  Divide/1 -> unit_vec/1
  vec_length/1(scaler) -> Divide/2

== system missile/missile/relative_motion/2x2 cross product/vec_normalize/vec_length ==
  vec : Inport
  Dot Product2 : DotProduct  InputSameDT=on  OutDataTypeStr=Inherit: Inherit via internal rule
  Sqrt1 : Sqrt  SaturateOnIntegerOverflow=on
  scaler : Outport
  wires:
  Sqrt1/1 -> scaler/1
  vec/1 -> Dot Product2/1, Dot Product2/2
  Dot Product2/1 -> Sqrt1/1

== system missile/missile/relative_motion/2x2 cross product/vec_normalize1/vec_length ==
  vec : Inport
  Dot Product2 : DotProduct  InputSameDT=on  OutDataTypeStr=Inherit: Inherit via internal rule
  Sqrt1 : Sqrt  SaturateOnIntegerOverflow=on
  scaler : Outport
  wires:
  Dot Product2/1 -> Sqrt1/1
  vec/1 -> Dot Product2/2, Dot Product2/1
  Sqrt1/1 -> scaler/1

== system missile/missile/relative_motion/2x2 cross product1/vec_normalize/vec_length ==
  vec : Inport
  Dot Product2 : DotProduct  InputSameDT=on  OutDataTypeStr=Inherit: Inherit via internal rule
  Sqrt1 : Sqrt  SaturateOnIntegerOverflow=on
  scaler : Outport
  wires:
  Dot Product2/1 -> Sqrt1/1
  vec/1 -> Dot Product2/2, Dot Product2/1
  Sqrt1/1 -> scaler/1

== system missile/missile/relative_motion/2x2 cross product1/vec_normalize1/vec_length ==
  vec : Inport
  Dot Product2 : DotProduct  InputSameDT=on  OutDataTypeStr=Inherit: Inherit via internal rule
  Sqrt1 : Sqrt  SaturateOnIntegerOverflow=on
  scaler : Outport
  wires:
  Sqrt1/1 -> scaler/1
  vec/1 -> Dot Product2/1, Dot Product2/2
  Dot Product2/1 -> Sqrt1/1

== system missile/missile/relative_motion/angle_offset/vec_normalize/vec_length ==
  vec : Inport
  Dot Product2 : DotProduct  InputSameDT=on  OutDataTypeStr=Inherit: Inherit via internal rule
  Sqrt1 : Sqrt  SaturateOnIntegerOverflow=on
  scaler : Outport
  wires:
  Sqrt1/1 -> scaler/1
  vec/1 -> Dot Product2/1, Dot Product2/2
  Dot Product2/1 -> Sqrt1/1

== system missile/missile/relative_motion/angle_offset/vec_normalize1/vec_length ==
  vec : Inport
  Dot Product2 : DotProduct  InputSameDT=on  OutDataTypeStr=Inherit: Inherit via internal rule
  Sqrt1 : Sqrt  SaturateOnIntegerOverflow=on
  scaler : Outport
  wires:
  Dot Product2/1 -> Sqrt1/1
  vec/1 -> Dot Product2/2, Dot Product2/1
  Sqrt1/1 -> scaler/1

== system missile/missile/relative_motion/angle_offset1/vec_normalize/vec_length ==
  vec : Inport
  Dot Product2 : DotProduct  InputSameDT=on  OutDataTypeStr=Inherit: Inherit via internal rule
  Sqrt1 : Sqrt  SaturateOnIntegerOverflow=on
  scaler : Outport
  wires:
  Dot Product2/1 -> Sqrt1/1
  vec/1 -> Dot Product2/2, Dot Product2/1
  Sqrt1/1 -> scaler/1

== system missile/missile/relative_motion/angle_offset1/vec_normalize1/vec_length ==
  vec : Inport
  Dot Product2 : DotProduct  InputSameDT=on  OutDataTypeStr=Inherit: Inherit via internal rule
  Sqrt1 : Sqrt  SaturateOnIntegerOverflow=on
  scaler : Outport
  wires:
  Sqrt1/1 -> scaler/1
  vec/1 -> Dot Product2/1, Dot Product2/2
  Dot Product2/1 -> Sqrt1/1

== matlab function missile/seeker/MATLAB Function1 ==
  settings: updateMethod=DISCRETE
  data: u input; hold output
function hold = signal_hold(u)
persistent active_signal;
if isempty(active_signal)
    active_signal = u;
elseif u==1
    active_signal = u;
end
hold = active_signal;

== matlab function missile/seeker/MATLAB Function ==
  settings: updateMethod=DISCRETE
  data: u input; hold output
function hold = signal_hold(u)
persistent active_signal;
if isempty(active_signal)
    active_signal = u;
elseif u==1
    active_signal = u;
end
hold = active_signal;

== matlab function missile/PNG/PNG ==
  data: dq_e input; K input; r_dot input; theta_v input; psi_v input; vm input; xe_m input; xe_t input; h input; TGO input; nn_req output size=1 3; time input; GP_switch input
function nn_req = png(dq_e, K, r_dot, theta_v, psi_v, vm, xe_m, xe_t, h, TGO, time, GP_switch)
g = 9.8;

%LOS angular velocity from e to traj
DCM_e2traj = [cos(theta_v)*cos(psi_v)  sin(theta_v)   -cos(theta_v)*sin(psi_v);
             -sin(theta_v)*cos(psi_v)  cos(theta_v)    sin(theta_v)*sin(psi_v);
              sin(psi_v)               0               cos(psi_v)];
dq_traj = DCM_e2traj*dq_e;

%normal load
if GP_switch > 0
    %throw trajectory parameter
    t_throw_end = 10;%s, ending time of throwing
    if TGO < 40
        t_throw_end = 1/5 * TGO;
    end
    if TGO > 150
        t_throw_end = 1/2 * t_throw_end;
        TGO = 80;
    end
    h_max = 25000;
    
    if time > t_throw_end
        dtheta_v = K*dq_traj(3);
        ny = abs(r_dot)*dtheta_v/g + cos(theta_v);
    else
        k = 1.5 * (h_max-h)/h_max;
        theta_delta = pi/6 * (1 - exp(-0.01*(30+TGO)));
        theta_pre = atan((xe_t(2)-xe_m(2)) / sqrt((xe_t(1)-xe_m(1))^2+(xe_t(3)-xe_m(3))^2));
        theta_opt = k * theta_delta + theta_pre;
        dtheta_v = pi/(2*t_throw_end) * theta_opt * sin(pi*time/t_throw_end);
        ny = abs(r_dot)*dtheta_v/g + cos(theta_v);
    end
else
    dtheta_v = K*dq_traj(3);
    ny = abs(r_dot)*dtheta_v/g + cos(theta_v);
end

dpsi_v = K*dq_traj(2);
nz = -abs(r_dot)*cos(theta_v)*dpsi_v/g;

nn_req = [0 ny nz];
end

== matlab function missile/target/MATLAB Function ==
  data: v input; ve output; theta input; psi input
function ve = v2ve(v, theta, psi)
vx = v * cos(theta) * cos(psi);      
vy = v * sin(theta);      
vz = -v * cos(theta) * sin(psi);
ve = [vx vy vz];
end

== matlab function missile/missile dynamics and kinematics/MATLAB Function ==
  data: v input; ve output; theta input; psi input
function ve = v2ve(v, theta, psi)
vx = v * cos(theta) * cos(psi);      
vy = v * sin(theta);      
vz = -v * cos(theta) * sin(psi);
ve = [vx vy vz];
end

== matlab function missile/PNG/MATLAB Function ==
  settings: updateMethod=DISCRETE
  data: r input; h input; TA input; ny_coe output; AO input
function ny_coe = fcn(r, h, TA, AO)
    persistent coe;
    if isempty(coe)
        TA_coe_max = 7; TA_coe_min = 2;
        AO_coe_max = 7; AO_coe_min = 2;
        r_coe_max = 7; r_coe_min = 2;
        h_coe_max = 3; h_coe_min = 2;
        AO_max = 60;%degree
        r_max = 80;  r_min = 20;%km
        h_max = 15; h_mid = 10; h_min = 5;%km
        n_max = 3;%g

        TA_abs = abs(rad2deg(TA));
        AO_abs = abs(rad2deg(AO));
        r = r / 1000.0;
        h = h / 1000.0;

        TA_coe = TA_coe_max - (TA_coe_max-TA_coe_min)/180*TA_abs;
        if AO_abs > AO_max
            AO_coe = AO_coe_max;
        else
            AO_coe = AO_coe_max - (AO_coe_max-AO_coe_min)/AO_max*AO_abs;
        end
        if r > r_max
            r_coe = r_coe_max;
        elseif r < r_min
            r_coe = r_coe_min;
        else
            r_coe = r_coe_max - (r_coe_max-r_coe_min)/(r_max-r_min)*(r_max-r);
        end
        if h >= h_min && h <= h_mid
            h_coe = h_coe_min + (h_coe_max-h_coe_min)/(h_mid-h_min)*(h-h_min);
        elseif h >= h_mid && h <= h_max
            h_coe = h_coe_max - (h_coe_max-h_coe_min)/(h_max-h_mid)*(h-h_mid);
        else
            h_coe = h_coe_min;
        end
        coe = n_max * (TA_coe+AO_coe+r_coe+h_coe) / (TA_coe_max+AO_coe_max+r_coe_max+h_coe_max);
    end
    
    ny_coe = coe;
end
